simulink model "Mmc"  (R2024b)
settings: Solver=ode23t  StartTime=0.0  StopTime=1  FixedStep=Ts_Power
values from neighbouring files (symbols this model uses):
  C_PM = 8e5    (= 800000)    [MmcParameters.m]    (also in MmcParameters_GFL.m = 0.006)
  Fnom = 50    [MmcParameters.m]    (also in MmcParameters_GFL.m)
  I_b = Snom/Vnom_AC/sqrt(3)    [MmcParameters.m]    (also in MmcParameters_GFL.m)
  Ipp_b = Snom/Vnom_AC/sqrt(3/2)    [MmcParameters.m]    (also in MmcParameters_GFL.m)
  kicir = R0*alpha_i    (= 17453.2925199)    [MmcParameters.m]    (also in MmcParameters_GFL.m = 523.598775598)
  kiout = R*alpha_i    (= 8726.64625997)    [MmcParameters.m]    (also in MmcParameters_GFL.m = 1308.996939)
  kip = alpha_p    (= 34906.5850399)    [MmcParameters.m]    (also in MmcParameters_GFL.m = 100)
  kpcir = L0*alpha_i    (= 2688.88888889)    [MmcParameters.m]    (also in MmcParameters_GFL.m = 66.6666666667)
  kpout = L*alpha_i    (= 1344.44444444)    [MmcParameters.m]    (also in MmcParameters_GFL.m = 166.666666667)
  kpp = alpha_p / alpha_i    (= 0.2)    [MmcParameters.m]    (also in MmcParameters_GFL.m = 0.00381971863421)
  L = L0/2    (= 0.00770309924565)    [MmcParameters.m]    (also in MmcParameters_GFL.m = 0.00636619772368)
  L0 = .2 * L_b    (= 0.0154061984913)    [MmcParameters.m]    (also in MmcParameters_GFL.m = 0.0127323954474)
  Lac = 32e-3    (= 0.032)    [MmcParameters.m]
  Nb_PM = 20    [MmcParameters.m]    (also in MmcParameters_GFL.m)
  R0 = .1    (= 0.1)    [MmcParameters.m]    (also in MmcParameters_GFL.m)
  Rac = 1    [MmcParameters.m]
  SCR = 2    [MmcParameters_GFL.m]
  SigmaM = 10    [MmcParameters_GFL.m]
  Snom = 80e6    (= 80000000)    [MmcParameters.m]    (also in MmcParameters_GFL.m)
  Ts_Power = 2e-6    (= 2e-06)    [MmcParameters.m]    (also in MmcParameters_GFL.m = 1e-05)
  V_b = Vnom_AC    (= 44000)    [MmcParameters.m]    (also in MmcParameters_GFL.m = 40000)
  VDCm = 80e3    (= 80000)    [MmcParameters.m]    (also in MmcParameters_GFL.m = 48000)
  VDCp = 80e3    (= 80000)    [MmcParameters.m]    (also in MmcParameters_GFL.m = 48000)
  Vnom_AC = 44e3    (= 44000)    [MmcParameters.m]    (also in MmcParameters_GFL.m = 40000)
  Vnom_PM = 4e3    (= 4000)    [MmcParameters.m]    (also in MmcParameters_GFL.m = 4800)
  w_b = 2*pi*Fnom    (= 314.159265359)    [MmcParameters.m]    (also in MmcParameters_GFL.m)
libraries: spsSeriesRLCBranchLib x8, spsCurrentMeasurementLib x7, spsHalfBridgeMMCLib x6, slpidlib x6, spsMeanLib x3, spsabctodq0Lib x3, spsDCVoltageSourceLib x2, spsdq0toabcLib x2, spsGroundLib x1, spsThreePhaseVIMeasurementLib x1, spsPLL3phLib x1, spsVoltageMeasurementLib x1
(part 1 of 2)
settings Model: Creator=The MathWorks, Inc.  LastModifiedBy=smile
settings SolverCC: AlgebraicLoopSolver=TrustRegion
settings DataIOCC: SaveFormat=StructureWithTime  SaveOutput=off  SignalLogging=off  DSMLogging=off  SaveTime=off  ReturnWorkspaceOutputs=off
settings OptimizationCC: ExpressionDepthLimit=2147483647  LifeSpan=inf
settings DebuggingCC: UnderspecifiedInitializationDetection=Classic  MergeDetectMultiDrivingBlocksExec=none  SolverPrmCheckMsg=warning  FcnCallInpInsideContextMsg=warning  UnconnectedInputMsg=warning  UnconnectedOutputMsg=warning  UnconnectedLineMsg=warning  AllowSymbolicDim=off  StateNameClashWarn=warning  SFUnexpectedBacktrackingDiag=warning  SFNoUnconditionalDefaultTransitionDiag=warning  SFExecutionAtInitializationDiag=none  ArithmeticOperatorsInVariantConditions=warning
settings HardwareCC: ProdBitPerPointer=32  ProdBitPerSizeT=32  ProdBitPerPtrDiffT=32  ProdLargestAtomicFloat=None  ProdIntDivRoundTo=Undefined  ProdEndianess=Unspecified  ProdWordSize=32  ProdHWDeviceType=32-bit Generic
settings ModelReferenceCC: EnableRefExpFcnMdlSchedulingChecks=on  PropagateSignalLabelsOutOfModel=off
settings SFSimCC: SimUseLocalCustomCode=off  CustomCodeUndefinedFunction=UseInterfaceOnly
settings RTWCC: RTWUseLocalCustomCode=off  GPUComputeCapability=3.5
settings CodeAppCC: StateflowObjectComments=on
settings GRTTargetCC: TargetLangStandard=C89/C90 (ANSI)  CombineOutputUpdateFcns=off  GRTInterface=on
settings ConfigComp: CovMetricSettings=dw  CovSaveCumulativeToWorkspaceVar=on  CovSaveSingleToWorkspaceVar=on  CovExternalEMLEnable=off
settings SimscapeCC: SimscapeNormalizeSystem=off  SimscapeNominalValues={1, 'bar'; 1, 'cm^3/s'; 1, 'bar*kg/s'; 1, 'kJ/kg'; 1, 'kW'; }

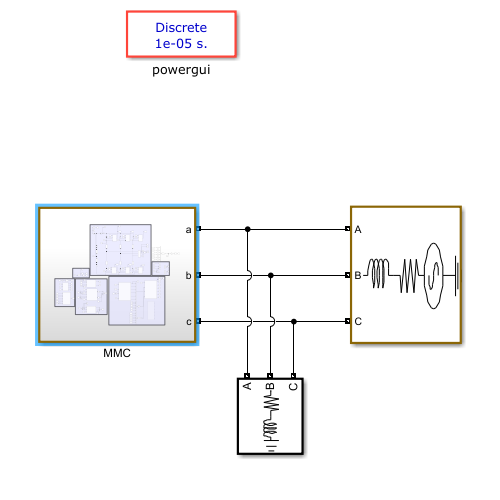
[thumbnail: Simulink's stored preview of the top-level diagram]
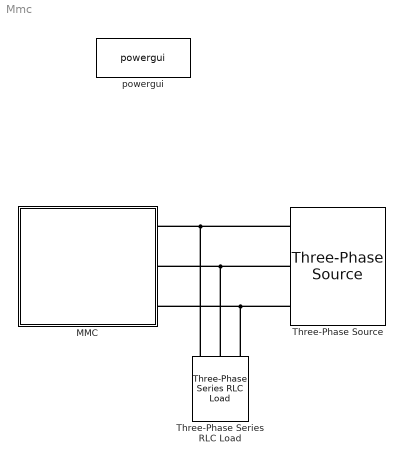
== system Mmc ==
  MMC : Subsystem
  Three-Phase Series RLC Load : spsThreePhaseSeriesRLCLoadLib/Three-Phase Series RLC Load  LConnTagsString=A|B|C  Configuration=Y (grounded)  NominalVoltage=Vnom_AC  Vabc=[1e3 1e3 1e3]  Vabcp=[1e3 1e3 1e3]  NominalFrequency=Fnom  UnbalancedPower=off  ActivePower=Snom/2  InductivePower=Snom/2  CapacitivePower=0  Pabc=[10e3 9e3 11e3]  QLabc=[100 90 110]  QCabc=[100 90 110]  Pabcp=[10e3 9e3 11e3]  QLabcp=[100 90 110]  QCabcp=[100 90 110]  Measurements=None  LoadType=constant Z
  Three-Phase Source : spsThreePhaseSourceLib/Three-Phase Source  InternalConnection=Yg  VoltagePhases=off  Voltage=Vnom_AC  PhaseAngle=0  Voltage_phases=[25e3 25e3 25e3]/sqrt(3)  PhaseAngles_phases=[0 -120 +120]  Frequency=50  NonIdealSource=on  SpecifyImpedance=on  Resistance=Rac/1e9  Inductance=Lac/1e4  ShortCircuitLevel=SCR*Snom  BaseVoltage=Vnom_AC  XRratio=7  BusType=swing  Pref=10e3  Qref=0  Prefabc=[10e3, 10e3, 10e3]  Qrefabc=[0, 0, 0]  Qmin=-inf  Qmax=inf
  powergui : sps_lib/powergui  Priority=1  SimulationMode=Discrete  SampleTime=Ts_Power  frequency=60  Iterations=50  frequencyindice=0  Pbase=100e6  ErrMax=1e-4  UnitsV=kV  UnitsW=MW  buscounter=0  FunctionMessages=off  echomessages=off  EnableUseOfTLC=off  CurrentSourceSwitches=off  DisableSnubberDevices=off  DisableRonSwitches=off  DisableVfSwitches=off  DisplayEquations=off  AutomaticDiscreteSolvers=off  SolverType=Tustin/Backward Euler (TBE)  Interpol=off  ExternalGateDelay=off  methode=off  Ts=10  x0status=blocks  SPID=off  SwTol=0  HookPort=off  NonlinearTolerance=1e-4  nMaxIteration=100  ContinueOnMaxIteration=off  RestoreLinks=warning  ResistiveCurrentMeasurement=off  Frange=[0:2:500]  Ylog=off  Xlog=on  ShowGrid=off  save=off  variable=ZData  structure=Vout  ZoomFFT=on  StartTime=0.15  cycles=2  DisplayStyle=1  fundamental=50  FreqAxis=on  MaxFrequency=6000  frequencyindicesteady=1  RmsSteady=1  display=off
  connections:
  Three-Phase Source/RConn1 -- Three-Phase Series RLC Load/LConn1 -- MMC/LConn1
  Three-Phase Source/RConn2 -- Three-Phase Series RLC Load/LConn2 -- MMC/LConn2
  Three-Phase Source/RConn3 -- Three-Phase Series RLC Load/LConn3 -- MMC/LConn3

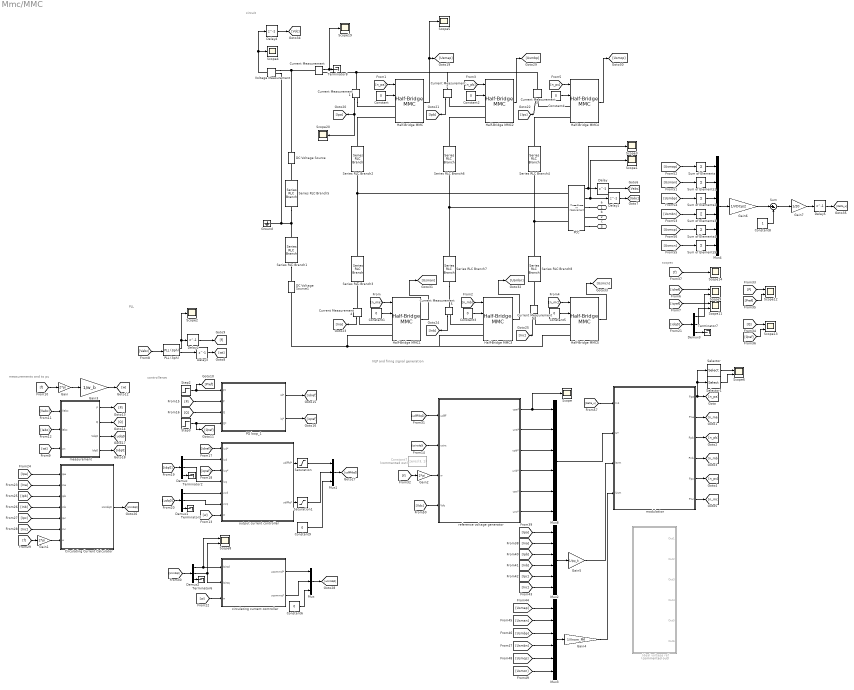
== system Mmc/MMC ==
  note: controllerws
  note: circuit
  note: scopes
  note: NLP and firing signal generation
  note: measurements and to pu
  note: PLL
  Circulating Current Calculator : Subsystem
  Constant{,1..6,9} (8 alike) : Constant  Value=0
  Constant7 : Constant  Commented=on  Value=zeros(3, 1)
  Constant8 : Constant
  Current Measurement{,1..6} (7 alike) : spsCurrentMeasurementLib/Current Measurement  PhasorSimulation=off  OutputType=Complex  PSBequivalent=0
  DC Voltage Source : spsDCVoltageSourceLib/DC Voltage Source  Amplitude=VDCp  Measurements=None
  DC Voltage Source1 : spsDCVoltageSourceLib/DC Voltage Source  Amplitude=VDCm  Measurements=None
  Delay{,1..3} (4 alike) : Delay  DelayLength=1  SampleTime=Ts_Power
  Delay4 : Delay  DelayLength=1  InputProcessing=Columns as channels (frame based)
  Delay5 : Delay  DelayLength=1  InputProcessing=Columns as channels (frame based)  SampleTime=Ts_Power
  Demux{,1..3} (4 alike) : Demux  Outputs=3
  Gain : Gain  Gain=2*pi
  Gain1 : Gain  Gain=2*pi
  Gain2 : Gain  Gain=2*pi
  Gain3 : Gain  Gain=1/w_b
  Gain4 : Gain  Gain=1/Vnom_PM
  Gain5 : Gain  Gain=1/Ipp_b
  Gain6 : Gain  Gain=1/VDCp/2
  Gain7 : Gain  Gain=1/20
  Ground : spsGroundLib/Ground  LConnTagsString=a
  Half-Bridge MMC{,1..5} (6 alike) : spsHalfBridgeMMCLib/Half-Bridge MMC  ModelType=Switching devices  n=Nb_PM  C=C_PM  Vc_Initial=Vc_Initial  Ron=Ron  Rs=Rs  Cs=Cs  Ron_Diode=1e-3  Rs_Diode=1e6  Cs_Diode=inf  Vf_Diode=1e-3  Rs_CurrentSource=inf  Ts=10e-6
      settings: LibrarySourceBlock=sps_lib/Power Electronics/Half-Bridge MMC
  Ideal voltage ref : Subsystem  Commented=on
  Mux : Mux  Inputs=3
  Mux1 : Mux  Inputs=3
  Mux{2..4,8} (4 alike) : Mux  Inputs=6
  PCC : spsThreePhaseVIMeasurementLib/Three-Phase V-I Measurement  VoltageMeasurement=phase-to-ground  SetLabelV=off  LabelV=Vabc  Vpu=on  VpuLL=off  CurrentMeasurement=yes  SetLabelI=off  LabelI=Iabc  Ipu=on  Pbase=Snom  Vbase=Vnom_AC  OutputType=Complex  PhasorSimulation=off  PSBequivalent=0
  PLL (3ph) : spsPLL3phLib/PLL (3ph)  Fmin=45  Par_Init=[0, 50]  ParK=[9.2/.2 (4.6/.2/.7)^2 0]  TcD=1e-4  MaxRateChangeFreq=12  FilterCutOffFreq=50  Ts=0  AGC=on
  PQ loop_1 : Subsystem
  Saturation : Saturate  UpperLimit=1.2  LowerLimit=-1.2
  Saturation1 : Saturate  UpperLimit=1.2  LowerLimit=-1.2
  Scope{,1..5,14,19..20} (9 alike) : Scope
  Scope{6,8..9,11..13} (6 alike) : Scope  NumInputPorts=2
  Selector : Selector  InputPortWidth=2*Nb_PM  IndexOptions=Index vector (dialog)  Indices=[1]  OutputSizes=1
  Selector1 : Selector  InputPortWidth=2*Nb_PM  IndexOptions=Index vector (dialog)  Indices=[Nb_PM]  OutputSizes=1
  Series RLC Branch{1..8} (8 alike) : spsSeriesRLCBranchLib/Series RLC Branch  LConnTagsString=__new0  RConnTagsString=__new0  BranchType=RL  Resistance=R0  Inductance=L0  SetiL0=off  InitialCurrent=0  Capacitance=1e-6  Setx0=off  InitialVoltage=0  Measurements=None
  Step2 : Step  Time=.3  Before=-.1  After=.7  SampleTime=Ts_Power
  Step3 : Step  Time=.7  Before=-.1  After=0.7  SampleTime=Ts_Power
  Sum : Sum  Inputs=|+-
  Sum of Elements{,1..5} (6 alike) : Sum  Inputs=+
  Terminator{2..3,6..8} (5 alike) : Terminator
  Voltage Measurement : spsVoltageMeasurementLib/Voltage Measurement  PhasorSimulation=off  OutputType=Complex  PSBequivalent=0
  circulating current controller : Subsystem
  measurement : Subsystem
  modulation : Subsystem
  output current controller : Subsystem
  reference voltage generator : Subsystem
  a : PMIOPort  Side=Left
  b : PMIOPort  Port=2  Side=Left
  c : PMIOPort  Port=3  Side=Left
  wires:
  Constant4/1 -> Half-Bridge MMC4/2
  [n_pc] -> Half-Bridge MMC4/1
  [n_pb] -> Half-Bridge MMC2/1
  [n_pa] -> Half-Bridge MMC/1
  [n_mb] -> Half-Bridge MMC3/1
  Constant1/1 -> Half-Bridge MMC1/2
  Constant3/1 -> Half-Bridge MMC3/2
  Half-Bridge MMC/1 -> Scope5/1, [Usmap]
  Constant2/1 -> Half-Bridge MMC2/2
  Constant/1 -> Half-Bridge MMC/2
  [n_ma] -> Half-Bridge MMC1/1
  Constant5/1 -> Half-Bridge MMC5/2
  [n_mc] -> Half-Bridge MMC5/1
  PCC/1 -> Scope3/1, Delay/1
  PCC/2 -> Scope1/1, Delay1/1
  [Vabc] -> measurement/1(Vabc)
  [Iabc] -> measurement/2(Iabc)
  [Vabc] -> PLL (3ph)/1
  PLL (3ph)/2 -> Delay3/1
  [wt] -> measurement/3(wt)
  PLL (3ph)/1 -> Scope2/1, Delay2/1
  [f] -> Gain/1
  Gain/1 -> Gain3/1
  Gain3/1 -> [w]
  [w] -> output current controller/7(w)
  circulating current controller/1(ucommd*) -> Mux/1
  circulating current controller/2(ucommq*) -> Mux/2
  Constant6/1 -> Mux/3
  measurement/1(P) -> [P]
  [idref] -> output current controller/1(ivd*)
  [iqref] -> output current controller/3(ivq*)
  measurement/3(Vdq0) -> [udq0]
  measurement/4(Idq0) -> [idq0]
  [idq0] -> Demux/1
  Demux/2 -> output current controller/4(ivq)
  Demux/1 -> output current controller/2(ivd)
  Demux/3 -> Terminator2/1
  [udq0] -> Demux1/1
  Demux1/1 -> output current controller/5(uvd)
  Demux1/2 -> output current controller/6(uvq)
  Demux1/3 -> Terminator3/1
  [w] -> circulating current controller/3(w)
  Current Measurement1/1 -> Scope20/1, [Ipa]
  Current Measurement2/1 -> [Ipb]
  Current Measurement3/1 -> [Ipc]
  Current Measurement4/1 -> [Ina]
  Current Measurement5/1 -> [Inb]
  Current Measurement6/1 -> [Inc]
  [Ipa] -> Circulating Current Calculator/1(ipa)
  [Ina] -> Circulating Current Calculator/2(ina)
  [Ipb] -> Circulating Current Calculator/3(ipb)
  [Inb] -> Circulating Current Calculator/4(inb)
  [Ipc] -> Circulating Current Calculator/5(ipc)
  [Inc] -> Circulating Current Calculator/6(inc)
  [f] -> Gain1/1
  Gain1/1 -> Circulating Current Calculator/7(w)
  Circulating Current Calculator/1(icircdq0) -> [Icircdq0]
  [Icircdq0] -> Demux2/1
  Demux2/1 -> Scope8/1, circulating current controller/1(Icircd)
  Demux2/2 -> circulating current controller/2(Icircq), Scope8/2
  Demux2/3 -> Terminator6/1
  Constant9/1 -> Mux1/3
  Mux1/1 -> [udiffdq0]
  Gain2/1 -> reference voltage generator/3(w)
  [f] -> Gain2/1
  measurement/2(Q) -> [Q]
  Step3/1 -> PQ loop_1/4(Q*), [Qref]
  Delay/1 -> [Vabc]
  Delay1/1 -> [Iabc]
  Delay2/1 -> [f]
  Delay3/1 -> [wt]
  modulation/1(Ppa) -> [n_pa], Selector1/1, Selector/1
  modulation/2(Pna) -> [n_ma]
  modulation/3(Ppb) -> [n_pb]
  modulation/4(Pnb) -> [n_mb]
  modulation/5(Ppc) -> [n_pc]
  modulation/6(Pnc) -> [n_mc]
  output current controller/1(udiffd*) -> Saturation/1
  Saturation/1 -> Mux1/1
  output current controller/2(udiffq*) -> Saturation1/1
  Saturation1/1 -> Mux1/2
  Step2/1 -> PQ loop_1/1(P*), [Pref]
  PQ loop_1/1(id*) -> [idref]
  PQ loop_1/2(iq*) -> [iqref]
  [idq0] -> Demux3/1
  Demux3/3 -> Terminator7/1
  [idref] -> Scope9/1
  Demux3/1 -> Scope9/2
  [iqref] -> Scope11/1
  Demux3/2 -> Scope11/2
  Mux/1 -> [ucircdq0]
  [P] -> Scope12/1
  [Pref] -> Scope12/2
  [Q] -> Scope13/1
  [Qref] -> Scope13/2
  [f] -> Scope14/1
  [P] -> PQ loop_1/2(P)
  [Q] -> PQ loop_1/3(Q)
  [udiffdq0] -> reference voltage generator/1(udiff)
  reference voltage generator/1(upa*) -> Scope/1, Mux8/1
  reference voltage generator/2(una*) -> Mux8/2
  reference voltage generator/3(upb*) -> Mux8/3
  reference voltage generator/4(unb*) -> Mux8/4
  reference voltage generator/5(upc*) -> Mux8/5
  reference voltage generator/6(unc*) -> Mux8/6
  [Ipa] -> Mux2/1
  [Ina] -> Mux2/2
  [Ipb] -> Mux2/3
  [Inb] -> Mux2/4
  [Ipc] -> Mux2/5
  [Inc] -> Mux2/6
  Mux2/1 -> Gain5/1
  Current Measurement/1 -> Scope19/1, Terminator8/1
  Half-Bridge MMC2/1 -> [Usmbp]
  Half-Bridge MMC4/1 -> [Usmcp]
  Half-Bridge MMC1/1 -> [Usman]
  Half-Bridge MMC3/1 -> [Usmbn]
  Half-Bridge MMC5/1 -> [Usmcn]
  [Usmap] -> Mux3/1
  [Usman] -> Mux3/2
  [Usmbp] -> Mux3/3
  [Usmbn] -> Mux3/4
  [Usmcp] -> Mux3/5
  Mux3/1 -> Gain4/1
  [Usmcn] -> Mux3/6
  Gain4/1 -> modulation/4(Usm)
  Gain5/1 -> modulation/3(Iarm)
  Selector/1 -> Scope6/1
  Selector1/1 -> Scope6/2
  Voltage Measurement/1 -> Delay4/1, Scope4/1
  Delay4/1 -> [Vdc]
  Mux8/1 -> modulation/2(U*)
  [Vdc] -> reference voltage generator/4(Vdc)
  [Usmap] -> Sum of Elements/1
  [Usman] -> Sum of Elements1/1
  [Usmbn] -> Sum of Elements3/1
  [Usmbp] -> Sum of Elements2/1
  [Usmcp] -> Sum of Elements4/1
  [Usmcn] -> Sum of Elements5/1
  Sum of Elements/1 -> Mux4/1
  Sum of Elements1/1 -> Mux4/2
  Sum of Elements2/1 -> Mux4/3
  Sum of Elements3/1 -> Mux4/4
  Sum of Elements4/1 -> Mux4/5
  Sum of Elements5/1 -> Mux4/6
  [Delta_u] -> modulation/1(In1)
  Mux4/1 -> Gain6/1
  Constant8/1 -> Sum/2
  Delay5/1 -> [Delta_u]
  Gain6/1 -> Sum/1
  Gain7/1 -> Delay5/1
  [ucircdq0] -> reference voltage generator/2(ucirc)
  Sum/1 -> Gain7/1
  connections:
  Series RLC Branch1/RConn1 -- DC Voltage Source1/RConn1
  Half-Bridge MMC5/LConn2 -- Half-Bridge MMC3/LConn2 -- Half-Bridge MMC1/LConn2 -- DC Voltage Source1/LConn1
  Series RLC Branch4/LConn1 -- Half-Bridge MMC4/LConn2
  Current Measurement/RConn1 -- Current Measurement2/LConn1 -- Current Measurement3/LConn1 -- Current Measurement1/LConn1
  Series RLC Branch8/LConn1 -- PCC/LConn3 -- Series RLC Branch4/RConn1
  Series RLC Branch1/LConn1 -- Series RLC Branch5/RConn1 -- Voltage Measurement/LConn2 -- Ground/LConn1
  Series RLC Branch2/LConn1 -- Half-Bridge MMC/LConn2
  Series RLC Branch3/LConn1 -- Series RLC Branch2/RConn1 -- PCC/LConn1
  Series RLC Branch6/LConn1 -- Half-Bridge MMC2/LConn2
  Series RLC Branch7/LConn1 -- Series RLC Branch6/RConn1 -- PCC/LConn2
  Series RLC Branch5/LConn1 -- DC Voltage Source/LConn1
  PCC/RConn1 -- a/RConn1
  b/RConn1 -- PCC/RConn2
  PCC/RConn3 -- c/RConn1
  Current Measurement/LConn1 -- DC Voltage Source/RConn1 -- Voltage Measurement/LConn1
  Current Measurement1/RConn1 -- Half-Bridge MMC/LConn1
  Half-Bridge MMC2/LConn1 -- Current Measurement2/RConn1
  Half-Bridge MMC4/LConn1 -- Current Measurement3/RConn1
  Half-Bridge MMC1/LConn1 -- Current Measurement4/RConn1
  Current Measurement4/LConn1 -- Series RLC Branch3/RConn1
  Series RLC Branch7/RConn1 -- Current Measurement5/LConn1
  Half-Bridge MMC3/LConn1 -- Current Measurement5/RConn1
  Current Measurement6/LConn1 -- Series RLC Branch8/RConn1
  Half-Bridge MMC5/LConn1 -- Current Measurement6/RConn1

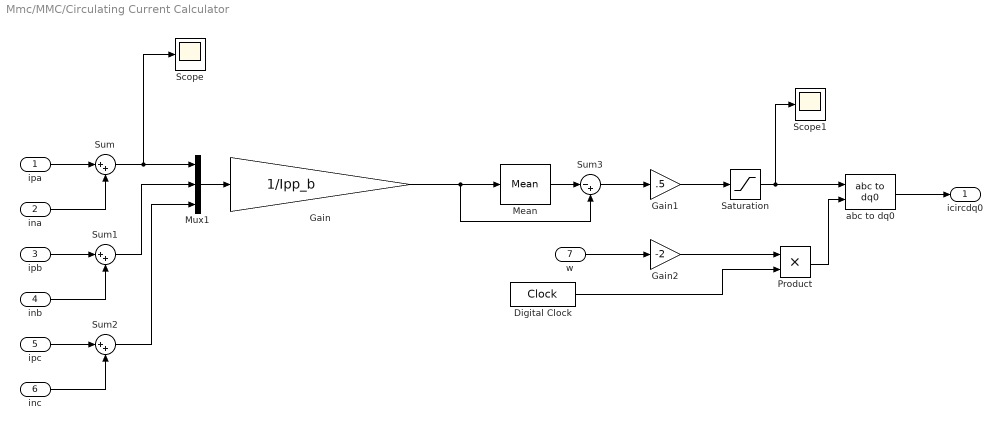
== system Mmc/MMC/Circulating Current Calculator ==
  ipa : Inport
  ina : Inport  Port=2
  ipb : Inport  Port=3
  inb : Inport  Port=4
  ipc : Inport  Port=5
  inc : Inport  Port=6
  w : Inport  Port=7
  Digital Clock : DigitalClock  SampleTime=Ts_Power
  Gain : Gain  Gain=1/Ipp_b
  Gain1 : Gain  Gain=.5
  Gain2 : Gain  Gain=-2
  Mean : spsMeanLib/Mean  Freq=Fnom*2*2  Vinit=0  Ts=Ts_Power
  Mux1 : Mux  Inputs=3
  Product : Product
  Saturation : Saturate  UpperLimit=1.2  LowerLimit=-1.2
  Scope : Scope
  Scope1 : Scope
  Sum : Sum  Inputs=|++
  Sum1 : Sum  Inputs=|++
  Sum2 : Sum  Inputs=|++
  Sum3 : Sum  Inputs=|-+
  abc to dq0 : spsabctodq0Lib/abc to dq0  Alignment=90 degrees behind phase A axis
  icircdq0 : Outport
  wires:
  Sum2/1 -> Mux1/3
  ina/1 -> Sum/2
  Mux1/1 -> Gain/1
  ipb/1 -> Sum1/1
  Sum/1 -> Scope/1, Mux1/1
  Sum1/1 -> Mux1/2
  ipc/1 -> Sum2/1
  inb/1 -> Sum1/2
  ipa/1 -> Sum/1
  inc/1 -> Sum2/2
  Gain1/1 -> Saturation/1
  abc to dq0/1 -> icircdq0/1
  w/1 -> Gain2/1
  Gain2/1 -> Product/1
  Digital Clock/1 -> Product/2
  Product/1 -> abc to dq0/2
  Mean/1 -> Sum3/1
  Sum3/1 -> Gain1/1
  Gain/1 -> Mean/1, Sum3/2
  Saturation/1 -> Scope1/1, abc to dq0/1

== system Mmc/MMC/Ideal voltage ref ==
  Gain4 : Gain  Gain=-1
  Gain5 : Gain  Gain=-1
  Gain6 : Gain  Gain=-1
  Sine Wave : Sin  Amplitude=sqrt(3/2)  Frequency=50*2*pi  SampleTime=Ts_Power
  Sine Wave1 : Sin  Amplitude=Vnom_AC*sqrt(2/3)/Vnom_PM/Nb_PM  Frequency=50*2*pi  Phase=4*pi/3  SampleTime=Ts_Power
  Sine Wave2 : Sin  Amplitude=Vnom_AC*sqrt(2/3)/Vnom_PM/Nb_PM  Frequency=50*2*pi  Phase=2*pi/3  SampleTime=Ts_Power
  Out1 : Outport
  Out2 : Outport  Port=2
  Out3 : Outport  Port=3
  Out4 : Outport  Port=4
  Out5 : Outport  Port=5
  Out6 : Outport  Port=6
  wires:
  Gain4/1 -> Out2/1
  Sine Wave1/1 -> Out3/1, Gain5/1
  Sine Wave2/1 -> Out5/1, Gain6/1
  Sine Wave/1 -> Out1/1, Gain4/1
  Gain6/1 -> Out6/1
  Gain5/1 -> Out4/1

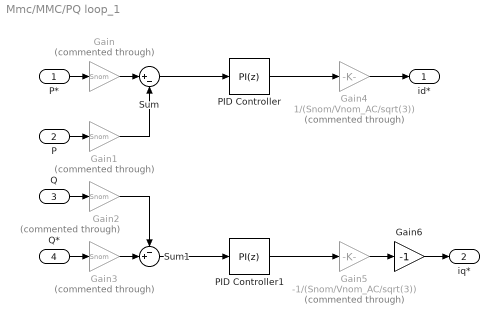
== system Mmc/MMC/PQ loop_1 ==
  P* : Inport
  P : Inport  Port=2
  Q : Inport  Port=3
  Q* : Inport  Port=4
  Gain{,1..3} (4 alike) : Gain  Commented=through  Gain=Snom
  Gain4 : Gain  Commented=through  Gain=1/(Snom/Vnom_AC/sqrt(3))
  Gain5 : Gain  Commented=through  Gain=-1/(Snom/Vnom_AC/sqrt(3))
  Gain6 : Gain  Gain=-1
  PID Controller : slpidlib/PID Controller  Controller=PI  Form=Parallel  TimeDomain=Discrete-time  UseExternalTs=off  SampleTime=-1  IntegratorMethod=Forward Euler  FilterMethod=Forward Euler  ControllerParametersSource=internal  P=kpp  I=kip  UseKiTs=off  D=0  UseExternalDerivativeSource=off  N=100  UseFilter=on  TunerSelectOption=Transfer Function Based (PID Tuner App)  InitialConditionSource=internal  InitialConditionForIntegrator=0  InitialConditionForFilter=0  DifferentiatorICPrevScaledInput=0  ExternalReset=none  TrackingMode=off  Kt=1  LimitOutput=off  SatLimitsSource=internal  UpperSaturationLimit=inf  LowerSaturationLimit=-inf  LinearizeAsGain=on  AntiWindupMode=none  Kb=1  LimitIntegrator=off  UpperIntegratorSaturationLimit=inf  LowerIntegratorSaturationLimit=-inf  POutMin=[]  POutMax=[]  IOutMin=[]  IOutMax=[]  DOutMin=[]  DOutMax=[]  NOutMin=[]  NOutMax=[]  SumOutMin=[]  SumOutMax=[]  SaturationOutMin=[]  SaturationOutMax=[]  PParamMin=[]  PParamMax=[]  IParamMin=[]  IParamMax=[]  DParamMin=[]  DParamMax=[]  NParamMin=[]  NParamMax=[]  KbParamMin=[]  KbParamMax=[]  KtParamMin=[]  KtParamMax=[]  KbOutMin=[]  KbOutMax=[]  KtOutMin=[]  KtOutMax=[]  IntegratorOutMin=[]  IntegratorOutMax=[]  FilterOutMin=[]  FilterOutMax=[]  SumI1OutMin=[]  SumI1OutMax=[]  SumI2OutMin=[]  SumI2OutMax=[]  SumI3OutMin=[]  SumI3OutMax=[]  SumI4OutMin=[]  SumI4OutMax=[]  SumDOutMin=[]  SumDOutMax=[]  DifferentiatorOutMin=[]  DifferentiatorOutMax=[]  FilterDiffOutCoefMin=[]  FilterDiffOutCoefMax=[]  ReciprocalOutMin=[]  ReciprocalOutMax=[]  SumDenOutMin=[]  SumDenOutMax=[]  SumNumOutMin=[]  SumNumOutMax=[]  DivideOutMin=[]  DivideOutMax=[]  UdiffTsProdOutMin=[]  UdiffTsProdOutMax=[]  NTsProdOutMin=[]  NTsProdOutMax=[]  UintegralTsProdOutMin=[]  UintegralTsProdOutMax=[]  UngainTsProdOutMin=[]  UngainTsProdOutMax=[]  ClampingZeroOutDataTypeStr=Inherit: Inherit via back propagation  ClampingZeroOutMin=[]  ClampingZeroOutMax=[]  FilterDenConstantOutDataTypeStr=Inherit: Inherit via back propagation  FilterDenConstantOutMin=[]  FilterDenConstantOutMax=[]  PCopyOutDataTypeStr=Inherit: Inherit via back propagation  PCopyOutMin=[]  PCopyOutMax=[]  NCopyOutDataTypeStr=Inherit: Inherit via back propagation  NCopyOutMin=[]  NCopyOutMax=[]  IntegratorContinuousStateAttributes=''  IntegratorStateMustResolveToSignalObject=off  IntegratorRTWStateStorageClass=Auto  FilterContinuousStateAttributes=''  FilterStateMustResolveToSignalObject=off  FilterRTWStateStorageClass=Auto  ParallelPVariant=InternalParameters  IdealPVariant=Disabled  IVariant=InternalParameters  DVariant=Disabled  IntegratorVariant=Discrete  SatVariant=Disabled  AWVariant=Passthrough  PCopyVariant=Disabled  TRVariant=Disabled  FdbkBlocksVariant=Forward  IdealPFdbkVariant=Disabled  SatFdbkVariant=Disabled  DerivativeFilterVariant=Disabled  NVariant=Disabled  NCopyVariant=Disabled_SignalSpec  FilterICVariant=Disabled  IntegratorICVariant=InternalICs  ExternalResetVariant=Disabled  TRSumVariant=Passthrough  SumFdbkVariant=Disabled  SumVariant=Sum_PI  TsampFilterVariant=InternalTs  TsampNgainVariant=Passthrough  TsampIntegralVariant=Disabled_SignalSpec  ExternalSaturationOutDataTypeStr=Inherit: Same as second input  DerivativeSourceVariant=Disabled  PreIntVariant=InternalPreInt
  PID Controller1 : slpidlib/PID Controller  Controller=PI  Form=Parallel  TimeDomain=Discrete-time  UseExternalTs=off  SampleTime=-1  IntegratorMethod=Forward Euler  FilterMethod=Forward Euler  ControllerParametersSource=internal  P=kpp  I=kip  UseKiTs=off  D=0  UseExternalDerivativeSource=off  N=100  UseFilter=on  TunerSelectOption=Transfer Function Based (PID Tuner App)  InitialConditionSource=internal  InitialConditionForIntegrator=0  InitialConditionForFilter=0  DifferentiatorICPrevScaledInput=0  ExternalReset=none  TrackingMode=off  Kt=1  LimitOutput=off  SatLimitsSource=internal  UpperSaturationLimit=inf  LowerSaturationLimit=-inf  LinearizeAsGain=on  AntiWindupMode=none  Kb=1  LimitIntegrator=off  UpperIntegratorSaturationLimit=inf  LowerIntegratorSaturationLimit=-inf  POutMin=[]  POutMax=[]  IOutMin=[]  IOutMax=[]  DOutMin=[]  DOutMax=[]  NOutMin=[]  NOutMax=[]  SumOutMin=[]  SumOutMax=[]  SaturationOutMin=[]  SaturationOutMax=[]  PParamMin=[]  PParamMax=[]  IParamMin=[]  IParamMax=[]  DParamMin=[]  DParamMax=[]  NParamMin=[]  NParamMax=[]  KbParamMin=[]  KbParamMax=[]  KtParamMin=[]  KtParamMax=[]  KbOutMin=[]  KbOutMax=[]  KtOutMin=[]  KtOutMax=[]  IntegratorOutMin=[]  IntegratorOutMax=[]  FilterOutMin=[]  FilterOutMax=[]  SumI1OutMin=[]  SumI1OutMax=[]  SumI2OutMin=[]  SumI2OutMax=[]  SumI3OutMin=[]  SumI3OutMax=[]  SumI4OutMin=[]  SumI4OutMax=[]  SumDOutMin=[]  SumDOutMax=[]  DifferentiatorOutMin=[]  DifferentiatorOutMax=[]  FilterDiffOutCoefMin=[]  FilterDiffOutCoefMax=[]  ReciprocalOutMin=[]  ReciprocalOutMax=[]  SumDenOutMin=[]  SumDenOutMax=[]  SumNumOutMin=[]  SumNumOutMax=[]  DivideOutMin=[]  DivideOutMax=[]  UdiffTsProdOutMin=[]  UdiffTsProdOutMax=[]  NTsProdOutMin=[]  NTsProdOutMax=[]  UintegralTsProdOutMin=[]  UintegralTsProdOutMax=[]  UngainTsProdOutMin=[]  UngainTsProdOutMax=[]  ClampingZeroOutDataTypeStr=Inherit: Inherit via back propagation  ClampingZeroOutMin=[]  ClampingZeroOutMax=[]  FilterDenConstantOutDataTypeStr=Inherit: Inherit via back propagation  FilterDenConstantOutMin=[]  FilterDenConstantOutMax=[]  PCopyOutDataTypeStr=Inherit: Inherit via back propagation  PCopyOutMin=[]  PCopyOutMax=[]  NCopyOutDataTypeStr=Inherit: Inherit via back propagation  NCopyOutMin=[]  NCopyOutMax=[]  IntegratorContinuousStateAttributes=''  IntegratorStateMustResolveToSignalObject=off  IntegratorRTWStateStorageClass=Auto  FilterContinuousStateAttributes=''  FilterStateMustResolveToSignalObject=off  FilterRTWStateStorageClass=Auto  ParallelPVariant=InternalParameters  IdealPVariant=Disabled  IVariant=InternalParameters  DVariant=Disabled  IntegratorVariant=Discrete  SatVariant=Disabled  AWVariant=Passthrough  PCopyVariant=Disabled  TRVariant=Disabled  FdbkBlocksVariant=Forward  IdealPFdbkVariant=Disabled  SatFdbkVariant=Disabled  DerivativeFilterVariant=Disabled  NVariant=Disabled  NCopyVariant=Disabled_SignalSpec  FilterICVariant=Disabled  IntegratorICVariant=InternalICs  ExternalResetVariant=Disabled  TRSumVariant=Passthrough  SumFdbkVariant=Disabled  SumVariant=Sum_PI  TsampFilterVariant=InternalTs  TsampNgainVariant=Passthrough  TsampIntegralVariant=Disabled_SignalSpec  ExternalSaturationOutDataTypeStr=Inherit: Same as second input  DerivativeSourceVariant=Disabled  PreIntVariant=InternalPreInt
  Sum : Sum  Inputs=|+-
  Sum1 : Sum  Inputs=-+|
  id* : Outport
  iq* : Outport  Port=2
  wires:
  P*/1 -> Gain/1
  P/1 -> Gain1/1
  Q*/1 -> Gain3/1
  Q/1 -> Gain2/1
  Sum/1 -> PID Controller/1
  Sum1/1 -> PID Controller1/1
  PID Controller/1 -> Gain4/1
  PID Controller1/1 -> Gain5/1
  Gain/1 -> Sum/1
  Gain1/1 -> Sum/2
  Gain2/1 -> Sum1/1
  Gain3/1 -> Sum1/2
  Gain4/1 -> id*/1
  Gain5/1 -> Gain6/1
  Gain6/1 -> iq*/1

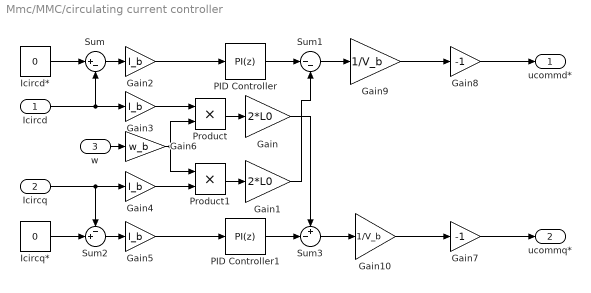
== system Mmc/MMC/circulating current controller ==
  Icircd : Inport
  Icircq : Inport  Port=2
  w : Inport  Port=3
  Gain : Gain  Gain=2*L0
  Gain1 : Gain  Gain=2*L0
  Gain10 : Gain  Gain=1/V_b
  Gain{2..5} (4 alike) : Gain  Gain=I_b
  Gain6 : Gain  Gain=w_b
  Gain7 : Gain  Gain=-1
  Gain8 : Gain  Gain=-1
  Gain9 : Gain  Gain=1/V_b
  Icircd* : Constant  Value=0
  Icircq* : Constant  Value=0
  PID Controller : slpidlib/PID Controller  Controller=PI  Form=Parallel  TimeDomain=Discrete-time  UseExternalTs=off  SampleTime=-1  IntegratorMethod=Forward Euler  FilterMethod=Forward Euler  ControllerParametersSource=internal  P=kpcir  I=kicir  UseKiTs=off  D=0  UseExternalDerivativeSource=off  N=100  UseFilter=on  TunerSelectOption=Transfer Function Based (PID Tuner App)  InitialConditionSource=internal  InitialConditionForIntegrator=0  InitialConditionForFilter=0  DifferentiatorICPrevScaledInput=0  ExternalReset=none  TrackingMode=off  Kt=1  LimitOutput=off  SatLimitsSource=internal  UpperSaturationLimit=inf  LowerSaturationLimit=-inf  LinearizeAsGain=on  AntiWindupMode=none  Kb=1  LimitIntegrator=off  UpperIntegratorSaturationLimit=inf  LowerIntegratorSaturationLimit=-inf  POutMin=[]  POutMax=[]  IOutMin=[]  IOutMax=[]  DOutMin=[]  DOutMax=[]  NOutMin=[]  NOutMax=[]  SumOutMin=[]  SumOutMax=[]  SaturationOutMin=[]  SaturationOutMax=[]  PParamMin=[]  PParamMax=[]  IParamMin=[]  IParamMax=[]  DParamMin=[]  DParamMax=[]  NParamMin=[]  NParamMax=[]  KbParamMin=[]  KbParamMax=[]  KtParamMin=[]  KtParamMax=[]  KbOutMin=[]  KbOutMax=[]  KtOutMin=[]  KtOutMax=[]  IntegratorOutMin=[]  IntegratorOutMax=[]  FilterOutMin=[]  FilterOutMax=[]  SumI1OutMin=[]  SumI1OutMax=[]  SumI2OutMin=[]  SumI2OutMax=[]  SumI3OutMin=[]  SumI3OutMax=[]  SumI4OutMin=[]  SumI4OutMax=[]  SumDOutMin=[]  SumDOutMax=[]  DifferentiatorOutMin=[]  DifferentiatorOutMax=[]  FilterDiffOutCoefMin=[]  FilterDiffOutCoefMax=[]  ReciprocalOutMin=[]  ReciprocalOutMax=[]  SumDenOutMin=[]  SumDenOutMax=[]  SumNumOutMin=[]  SumNumOutMax=[]  DivideOutMin=[]  DivideOutMax=[]  UdiffTsProdOutMin=[]  UdiffTsProdOutMax=[]  NTsProdOutMin=[]  NTsProdOutMax=[]  UintegralTsProdOutMin=[]  UintegralTsProdOutMax=[]  UngainTsProdOutMin=[]  UngainTsProdOutMax=[]  ClampingZeroOutDataTypeStr=Inherit: Inherit via back propagation  ClampingZeroOutMin=[]  ClampingZeroOutMax=[]  FilterDenConstantOutDataTypeStr=Inherit: Inherit via back propagation  FilterDenConstantOutMin=[]  FilterDenConstantOutMax=[]  PCopyOutDataTypeStr=Inherit: Inherit via back propagation  PCopyOutMin=[]  PCopyOutMax=[]  NCopyOutDataTypeStr=Inherit: Inherit via back propagation  NCopyOutMin=[]  NCopyOutMax=[]  IntegratorContinuousStateAttributes=''  IntegratorStateMustResolveToSignalObject=off  IntegratorRTWStateStorageClass=Auto  FilterContinuousStateAttributes=''  FilterStateMustResolveToSignalObject=off  FilterRTWStateStorageClass=Auto  ParallelPVariant=InternalParameters  IdealPVariant=Disabled  IVariant=InternalParameters  DVariant=Disabled  IntegratorVariant=Discrete  SatVariant=Disabled  AWVariant=Passthrough  PCopyVariant=Disabled  TRVariant=Disabled  FdbkBlocksVariant=Forward  IdealPFdbkVariant=Disabled  SatFdbkVariant=Disabled  DerivativeFilterVariant=Disabled  NVariant=Disabled  NCopyVariant=Disabled_SignalSpec  FilterICVariant=Disabled  IntegratorICVariant=InternalICs  ExternalResetVariant=Disabled  TRSumVariant=Passthrough  SumFdbkVariant=Disabled  SumVariant=Sum_PI  TsampFilterVariant=InternalTs  TsampNgainVariant=Passthrough  TsampIntegralVariant=Disabled_SignalSpec  ExternalSaturationOutDataTypeStr=Inherit: Same as second input  DerivativeSourceVariant=Disabled  PreIntVariant=InternalPreInt
  PID Controller1 : slpidlib/PID Controller  Controller=PI  Form=Parallel  TimeDomain=Discrete-time  UseExternalTs=off  SampleTime=-1  IntegratorMethod=Forward Euler  FilterMethod=Forward Euler  ControllerParametersSource=internal  P=kpcir  I=kicir  UseKiTs=off  D=0  UseExternalDerivativeSource=off  N=100  UseFilter=on  TunerSelectOption=Transfer Function Based (PID Tuner App)  InitialConditionSource=internal  InitialConditionForIntegrator=0  InitialConditionForFilter=0  DifferentiatorICPrevScaledInput=0  ExternalReset=none  TrackingMode=off  Kt=1  LimitOutput=off  SatLimitsSource=internal  UpperSaturationLimit=inf  LowerSaturationLimit=-inf  LinearizeAsGain=on  AntiWindupMode=none  Kb=1  LimitIntegrator=off  UpperIntegratorSaturationLimit=inf  LowerIntegratorSaturationLimit=-inf  POutMin=[]  POutMax=[]  IOutMin=[]  IOutMax=[]  DOutMin=[]  DOutMax=[]  NOutMin=[]  NOutMax=[]  SumOutMin=[]  SumOutMax=[]  SaturationOutMin=[]  SaturationOutMax=[]  PParamMin=[]  PParamMax=[]  IParamMin=[]  IParamMax=[]  DParamMin=[]  DParamMax=[]  NParamMin=[]  NParamMax=[]  KbParamMin=[]  KbParamMax=[]  KtParamMin=[]  KtParamMax=[]  KbOutMin=[]  KbOutMax=[]  KtOutMin=[]  KtOutMax=[]  IntegratorOutMin=[]  IntegratorOutMax=[]  FilterOutMin=[]  FilterOutMax=[]  SumI1OutMin=[]  SumI1OutMax=[]  SumI2OutMin=[]  SumI2OutMax=[]  SumI3OutMin=[]  SumI3OutMax=[]  SumI4OutMin=[]  SumI4OutMax=[]  SumDOutMin=[]  SumDOutMax=[]  DifferentiatorOutMin=[]  DifferentiatorOutMax=[]  FilterDiffOutCoefMin=[]  FilterDiffOutCoefMax=[]  ReciprocalOutMin=[]  ReciprocalOutMax=[]  SumDenOutMin=[]  SumDenOutMax=[]  SumNumOutMin=[]  SumNumOutMax=[]  DivideOutMin=[]  DivideOutMax=[]  UdiffTsProdOutMin=[]  UdiffTsProdOutMax=[]  NTsProdOutMin=[]  NTsProdOutMax=[]  UintegralTsProdOutMin=[]  UintegralTsProdOutMax=[]  UngainTsProdOutMin=[]  UngainTsProdOutMax=[]  ClampingZeroOutDataTypeStr=Inherit: Inherit via back propagation  ClampingZeroOutMin=[]  ClampingZeroOutMax=[]  FilterDenConstantOutDataTypeStr=Inherit: Inherit via back propagation  FilterDenConstantOutMin=[]  FilterDenConstantOutMax=[]  PCopyOutDataTypeStr=Inherit: Inherit via back propagation  PCopyOutMin=[]  PCopyOutMax=[]  NCopyOutDataTypeStr=Inherit: Inherit via back propagation  NCopyOutMin=[]  NCopyOutMax=[]  IntegratorContinuousStateAttributes=''  IntegratorStateMustResolveToSignalObject=off  IntegratorRTWStateStorageClass=Auto  FilterContinuousStateAttributes=''  FilterStateMustResolveToSignalObject=off  FilterRTWStateStorageClass=Auto  ParallelPVariant=InternalParameters  IdealPVariant=Disabled  IVariant=InternalParameters  DVariant=Disabled  IntegratorVariant=Discrete  SatVariant=Disabled  AWVariant=Passthrough  PCopyVariant=Disabled  TRVariant=Disabled  FdbkBlocksVariant=Forward  IdealPFdbkVariant=Disabled  SatFdbkVariant=Disabled  DerivativeFilterVariant=Disabled  NVariant=Disabled  NCopyVariant=Disabled_SignalSpec  FilterICVariant=Disabled  IntegratorICVariant=InternalICs  ExternalResetVariant=Disabled  TRSumVariant=Passthrough  SumFdbkVariant=Disabled  SumVariant=Sum_PI  TsampFilterVariant=InternalTs  TsampNgainVariant=Passthrough  TsampIntegralVariant=Disabled_SignalSpec  ExternalSaturationOutDataTypeStr=Inherit: Same as second input  DerivativeSourceVariant=Disabled  PreIntVariant=InternalPreInt
  Product : Product
  Product1 : Product
  Sum : Sum  Inputs=|+-
  Sum1 : Sum  Inputs=|--
  Sum2 : Sum  Inputs=-+|
  Sum3 : Sum  Inputs=+-|
  ucommd* : Outport
  ucommq* : Outport  Port=2
  wires:
  Icircd*/1 -> Sum/1
  Sum/1 -> Gain2/1
  Icircd/1 -> Gain3/1, Sum/2
  Icircq/1 -> Gain4/1, Sum2/1
  Icircq*/1 -> Sum2/2
  Sum2/1 -> Gain5/1
  PID Controller1/1 -> Sum3/2
  PID Controller/1 -> Sum1/1
  w/1 -> Gain6/1
  Product/1 -> Gain/1
  Product1/1 -> Gain1/1
  Sum1/1 -> Gain9/1
  Sum3/1 -> Gain10/1
  Gain/1 -> Sum3/1
  Gain1/1 -> Sum1/2
  Gain2/1 -> PID Controller/1
  Gain3/1 -> Product/1
  Gain6/1 -> Product1/1, Product/2
  Gain4/1 -> Product1/2
  Gain5/1 -> PID Controller1/1
  Gain9/1 -> Gain8/1
  Gain10/1 -> Gain7/1
  Gain8/1 -> ucommd*/1
  Gain7/1 -> ucommq*/1

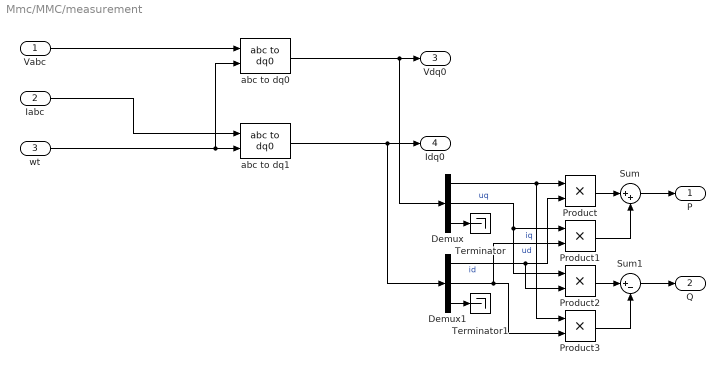
== system Mmc/MMC/measurement ==
  Vabc : Inport
  Iabc : Inport  Port=2
  wt : Inport  Port=3
  Demux : Demux  Outputs=3
  Demux1 : Demux  Outputs=3
  Product{,1..3} (4 alike) : Product
  Sum : Sum  Inputs=|++
  Sum1 : Sum  Inputs=|+-
  Terminator : Terminator
  Terminator1 : Terminator
  abc to dq0 : spsabctodq0Lib/abc to dq0  Alignment=90 degrees behind phase A axis
  abc to dq1 : spsabctodq0Lib/abc to dq0  Alignment=90 degrees behind phase A axis
  P : Outport
  Q : Outport  Port=2
  Vdq0 : Outport  Port=3
  Idq0 : Outport  Port=4
  wires:
  wt/1 -> abc to dq0/2, abc to dq1/2
  Vabc/1 -> abc to dq0/1
  Iabc/1 -> abc to dq1/1
  Demux/3 -> Terminator/1
  Demux1/3 -> Terminator1/1
  Demux/1 -> Product3/1, Product/1  "ud"
  Demux/2 -> Product1/1, Product2/1  "uq"
  Demux1/2 -> Product1/2, Product3/2  "iq"
  Product/1 -> Sum/1
  Product1/1 -> Sum/2
  Product2/1 -> Sum1/1
  Product3/1 -> Sum1/2
  Demux1/1 -> Product2/2, Product/2  "id"
  abc to dq0/1 -> Demux/1, Vdq0/1
  abc to dq1/1 -> Demux1/1, Idq0/1
  Sum/1 -> P/1
  Sum1/1 -> Q/1

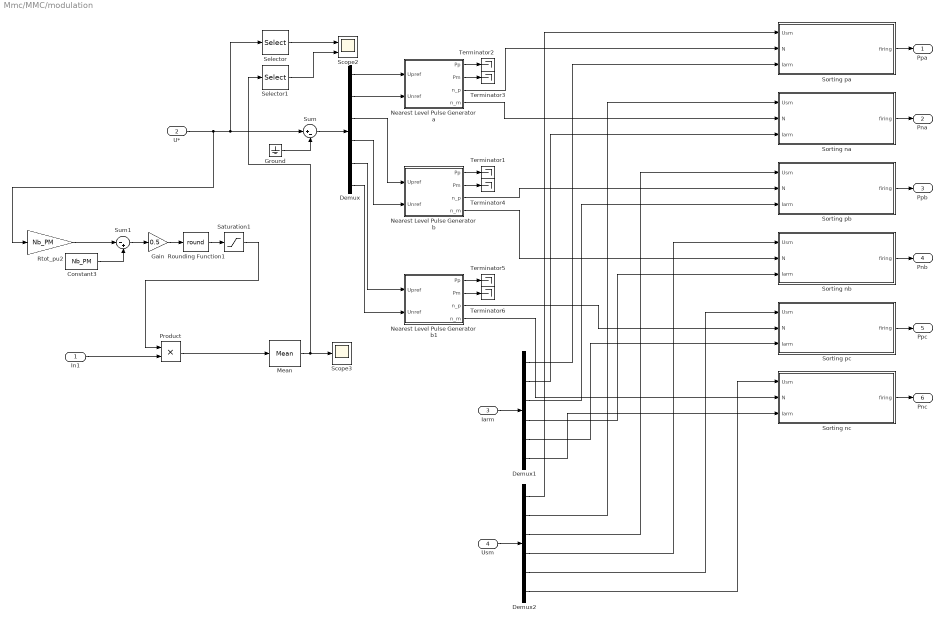
== system Mmc/MMC/modulation ==
  In1 : Inport
  U* : Inport  Port=2
  Iarm : Inport  Port=3
  Usm : Inport  Port=4
  Constant3 : Constant  Value=Nb_PM
  Demux : Demux  Outputs=6
  Demux1 : Demux  Outputs=6
  Demux2 : Demux  Outputs=6
  Gain : Gain  Gain=0.5
  Ground : Ground
  Mean : spsMeanLib/Mean  Freq=Fnom*2  Vinit=0  Ts=Ts_Power
  "Nearest Level Pulse Generator a " : Subsystem
  Nearest Level Pulse Generator b : Subsystem
  Nearest Level Pulse Generator b1 : Subsystem
  Product : Product
  Rounding Function1 : Rounding  Operator=round
  Rtot_pu2 : Gain  Gain=Nb_PM  SaturateOnIntegerOverflow=on  OutDataTypeStr=Inherit: Same as input  ParamDataTypeStr=Inherit: Same as input
  Saturation1 : Saturate  UpperLimit=Nb_PM  LowerLimit=0
  Scope2 : Scope  NumInputPorts=2
  Scope3 : Scope
  Selector : Selector  InputPortWidth=6  IndexOptions=Index vector (dialog)  Indices=[1]  OutputSizes=1
  Selector1 : Selector  InputPortWidth=6  IndexOptions=Index vector (dialog)  Indices=[1]  OutputSizes=1
  Sorting na : Subsystem
  Sorting nb : Subsystem
  Sorting nc : Subsystem
  Sorting pa : Subsystem
  Sorting pb : Subsystem
  Sorting pc : Subsystem
  Sum : Sum  Inputs=|+-
  Sum1 : Sum  Inputs=|-+
  Terminator{1..6} (6 alike) : Terminator
  Ppa : Outport
  Pna : Outport  Port=2
  Ppb : Outport  Port=3
  Pnb : Outport  Port=4
  Ppc : Outport  Port=5
  Pnc : Outport  Port=6
  wires:
  Demux/1 -> "Nearest Level Pulse Generator a "/1(Upref)
  "Nearest Level Pulse Generator a "/3(n_p) -> Sorting pa/2(N)
  "Nearest Level Pulse Generator a "/4(n_m) -> Sorting na/2(N)
  Demux/2 -> "Nearest Level Pulse Generator a "/2(Unref)
  Demux/4 -> Nearest Level Pulse Generator b/2(Unref)
  Demux/3 -> Nearest Level Pulse Generator b/1(Upref)
  Demux/6 -> Nearest Level Pulse Generator b1/2(Unref)
  Demux/5 -> Nearest Level Pulse Generator b1/1(Upref)
  Sorting pa/1(firing) -> Ppa/1
  Sorting na/1(firing) -> Pna/1
  "Nearest Level Pulse Generator a "/1(Pp) -> Terminator2/1
  "Nearest Level Pulse Generator a "/2(Pm) -> Terminator3/1
  Sorting pb/1(firing) -> Ppb/1
  Sorting nb/1(firing) -> Pnb/1
  Nearest Level Pulse Generator b/3(n_p) -> Sorting pb/2(N)
  Nearest Level Pulse Generator b/4(n_m) -> Sorting nb/2(N)
  Nearest Level Pulse Generator b/1(Pp) -> Terminator1/1
  Nearest Level Pulse Generator b/2(Pm) -> Terminator4/1
  Sorting nc/1(firing) -> Pnc/1
  Sorting pc/1(firing) -> Ppc/1
  Nearest Level Pulse Generator b1/3(n_p) -> Sorting pc/2(N)
  Nearest Level Pulse Generator b1/4(n_m) -> Sorting nc/2(N)
  Iarm/1 -> Demux1/1
  Demux1/1 -> Sorting pa/3(Iarm)
  Demux1/2 -> Sorting na/3(Iarm)
  Demux1/3 -> Sorting pb/3(Iarm)
  Demux1/4 -> Sorting nb/3(Iarm)
  Demux1/5 -> Sorting pc/3(Iarm)
  Demux1/6 -> Sorting nc/3(Iarm)
  Usm/1 -> Demux2/1
  Demux2/6 -> Sorting nc/1(Usm)
  Demux2/5 -> Sorting pc/1(Usm)
  Demux2/4 -> Sorting nb/1(Usm)
  Demux2/3 -> Sorting pb/1(Usm)
  Demux2/2 -> Sorting na/1(Usm)
  Demux2/1 -> Sorting pa/1(Usm)
  Nearest Level Pulse Generator b1/1(Pp) -> Terminator5/1
  Nearest Level Pulse Generator b1/2(Pm) -> Terminator6/1
  Sum/1 -> Demux/1
  In1/1 -> Product/2
  Product/1 -> Mean/1
  Mean/1 -> Selector1/1, Scope3/1
  U*/1 -> Rtot_pu2/1, Selector/1, Sum/1
  Sum1/1 -> Gain/1
  Constant3/1 -> Sum1/2
  Gain/1 -> Rounding Function1/1
  Rtot_pu2/1 -> Sum1/1
  Rounding Function1/1 -> Saturation1/1
  Saturation1/1 -> Product/1
  Selector/1 -> Scope2/1
  Selector1/1 -> Scope2/2
  Ground/1 -> Sum/2

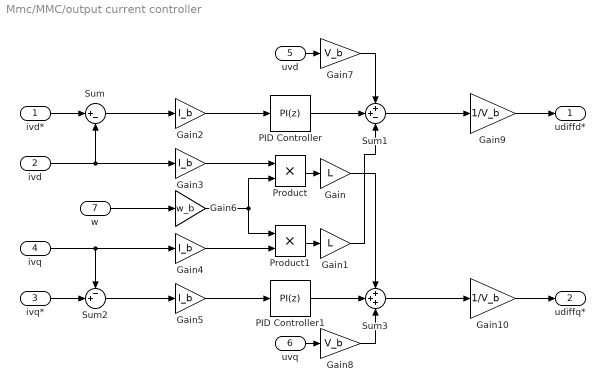
== system Mmc/MMC/output current controller ==
  ivd* : Inport
  ivd : Inport  Port=2
  ivq* : Inport  Port=3
  ivq : Inport  Port=4
  uvd : Inport  Port=5
  uvq : Inport  Port=6
  w : Inport  Port=7
  Gain : Gain  Gain=L
  Gain1 : Gain  Gain=L
  Gain10 : Gain  Gain=1/V_b
  Gain{2..5} (4 alike) : Gain  Gain=I_b
  Gain6 : Gain  Gain=w_b
  Gain7 : Gain  Gain=V_b
  Gain8 : Gain  Gain=V_b
  Gain9 : Gain  Gain=1/V_b
  PID Controller : slpidlib/PID Controller  Controller=PI  Form=Parallel  TimeDomain=Discrete-time  UseExternalTs=off  SampleTime=-1  IntegratorMethod=Forward Euler  FilterMethod=Forward Euler  ControllerParametersSource=internal  P=kpout  I=kiout  UseKiTs=off  D=0  UseExternalDerivativeSource=off  N=100  UseFilter=on  TunerSelectOption=Transfer Function Based (PID Tuner App)  InitialConditionSource=internal  InitialConditionForIntegrator=0  InitialConditionForFilter=0  DifferentiatorICPrevScaledInput=0  ExternalReset=none  TrackingMode=off  Kt=1  LimitOutput=off  SatLimitsSource=internal  UpperSaturationLimit=Vnom_AC  LowerSaturationLimit=-Vnom_AC  LinearizeAsGain=on  AntiWindupMode=clamping  Kb=1  LimitIntegrator=off  UpperIntegratorSaturationLimit=inf  LowerIntegratorSaturationLimit=-inf  POutMin=[]  POutMax=[]  IOutMin=[]  IOutMax=[]  DOutMin=[]  DOutMax=[]  NOutMin=[]  NOutMax=[]  SumOutMin=[]  SumOutMax=[]  SaturationOutMin=[]  SaturationOutMax=[]  PParamMin=[]  PParamMax=[]  IParamMin=[]  IParamMax=[]  DParamMin=[]  DParamMax=[]  NParamMin=[]  NParamMax=[]  KbParamMin=[]  KbParamMax=[]  KtParamMin=[]  KtParamMax=[]  KbOutMin=[]  KbOutMax=[]  KtOutMin=[]  KtOutMax=[]  IntegratorOutMin=[]  IntegratorOutMax=[]  FilterOutMin=[]  FilterOutMax=[]  SumI1OutMin=[]  SumI1OutMax=[]  SumI2OutMin=[]  SumI2OutMax=[]  SumI3OutMin=[]  SumI3OutMax=[]  SumI4OutMin=[]  SumI4OutMax=[]  SumDOutMin=[]  SumDOutMax=[]  DifferentiatorOutMin=[]  DifferentiatorOutMax=[]  FilterDiffOutCoefMin=[]  FilterDiffOutCoefMax=[]  ReciprocalOutMin=[]  ReciprocalOutMax=[]  SumDenOutMin=[]  SumDenOutMax=[]  SumNumOutMin=[]  SumNumOutMax=[]  DivideOutMin=[]  DivideOutMax=[]  UdiffTsProdOutMin=[]  UdiffTsProdOutMax=[]  NTsProdOutMin=[]  NTsProdOutMax=[]  UintegralTsProdOutMin=[]  UintegralTsProdOutMax=[]  UngainTsProdOutMin=[]  UngainTsProdOutMax=[]  ClampingZeroOutDataTypeStr=Inherit: Inherit via back propagation  ClampingZeroOutMin=[]  ClampingZeroOutMax=[]  FilterDenConstantOutDataTypeStr=Inherit: Inherit via back propagation  FilterDenConstantOutMin=[]  FilterDenConstantOutMax=[]  PCopyOutDataTypeStr=Inherit: Inherit via back propagation  PCopyOutMin=[]  PCopyOutMax=[]  NCopyOutDataTypeStr=Inherit: Inherit via back propagation  NCopyOutMin=[]  NCopyOutMax=[]  IntegratorContinuousStateAttributes=''  IntegratorStateMustResolveToSignalObject=off  IntegratorRTWStateStorageClass=Auto  FilterContinuousStateAttributes=''  FilterStateMustResolveToSignalObject=off  FilterRTWStateStorageClass=Auto  ParallelPVariant=InternalParameters  IdealPVariant=Disabled  IVariant=InternalParameters  DVariant=Disabled  IntegratorVariant=Discrete  SatVariant=Disabled  AWVariant=Passthrough  PCopyVariant=Disabled  TRVariant=Disabled  FdbkBlocksVariant=Forward  IdealPFdbkVariant=Disabled  SatFdbkVariant=Disabled  DerivativeFilterVariant=Disabled  NVariant=Disabled  NCopyVariant=Disabled_SignalSpec  FilterICVariant=Disabled  IntegratorICVariant=InternalICs  ExternalResetVariant=Disabled  TRSumVariant=Passthrough  SumFdbkVariant=Disabled  SumVariant=Sum_PI  TsampFilterVariant=InternalTs  TsampNgainVariant=Passthrough  TsampIntegralVariant=Disabled_SignalSpec  ExternalSaturationOutDataTypeStr=Inherit: Same as second input  DerivativeSourceVariant=Disabled  PreIntVariant=InternalPreInt
  PID Controller1 : slpidlib/PID Controller  Controller=PI  Form=Parallel  TimeDomain=Discrete-time  UseExternalTs=off  SampleTime=-1  IntegratorMethod=Forward Euler  FilterMethod=Forward Euler  ControllerParametersSource=internal  P=kpout  I=kiout  UseKiTs=off  D=0  UseExternalDerivativeSource=off  N=100  UseFilter=on  TunerSelectOption=Transfer Function Based (PID Tuner App)  InitialConditionSource=internal  InitialConditionForIntegrator=0  InitialConditionForFilter=0  DifferentiatorICPrevScaledInput=0  ExternalReset=none  TrackingMode=off  Kt=1  LimitOutput=off  SatLimitsSource=internal  UpperSaturationLimit=Vnom_AC  LowerSaturationLimit=-Vnom_AC  LinearizeAsGain=on  AntiWindupMode=clamping  Kb=1  LimitIntegrator=off  UpperIntegratorSaturationLimit=inf  LowerIntegratorSaturationLimit=-inf  POutMin=[]  POutMax=[]  IOutMin=[]  IOutMax=[]  DOutMin=[]  DOutMax=[]  NOutMin=[]  NOutMax=[]  SumOutMin=[]  SumOutMax=[]  SaturationOutMin=[]  SaturationOutMax=[]  PParamMin=[]  PParamMax=[]  IParamMin=[]  IParamMax=[]  DParamMin=[]  DParamMax=[]  NParamMin=[]  NParamMax=[]  KbParamMin=[]  KbParamMax=[]  KtParamMin=[]  KtParamMax=[]  KbOutMin=[]  KbOutMax=[]  KtOutMin=[]  KtOutMax=[]  IntegratorOutMin=[]  IntegratorOutMax=[]  FilterOutMin=[]  FilterOutMax=[]  SumI1OutMin=[]  SumI1OutMax=[]  SumI2OutMin=[]  SumI2OutMax=[]  SumI3OutMin=[]  SumI3OutMax=[]  SumI4OutMin=[]  SumI4OutMax=[]  SumDOutMin=[]  SumDOutMax=[]  DifferentiatorOutMin=[]  DifferentiatorOutMax=[]  FilterDiffOutCoefMin=[]  FilterDiffOutCoefMax=[]  ReciprocalOutMin=[]  ReciprocalOutMax=[]  SumDenOutMin=[]  SumDenOutMax=[]  SumNumOutMin=[]  SumNumOutMax=[]  DivideOutMin=[]  DivideOutMax=[]  UdiffTsProdOutMin=[]  UdiffTsProdOutMax=[]  NTsProdOutMin=[]  NTsProdOutMax=[]  UintegralTsProdOutMin=[]  UintegralTsProdOutMax=[]  UngainTsProdOutMin=[]  UngainTsProdOutMax=[]  ClampingZeroOutDataTypeStr=Inherit: Inherit via back propagation  ClampingZeroOutMin=[]  ClampingZeroOutMax=[]  FilterDenConstantOutDataTypeStr=Inherit: Inherit via back propagation  FilterDenConstantOutMin=[]  FilterDenConstantOutMax=[]  PCopyOutDataTypeStr=Inherit: Inherit via back propagation  PCopyOutMin=[]  PCopyOutMax=[]  NCopyOutDataTypeStr=Inherit: Inherit via back propagation  NCopyOutMin=[]  NCopyOutMax=[]  IntegratorContinuousStateAttributes=''  IntegratorStateMustResolveToSignalObject=off  IntegratorRTWStateStorageClass=Auto  FilterContinuousStateAttributes=''  FilterStateMustResolveToSignalObject=off  FilterRTWStateStorageClass=Auto  ParallelPVariant=InternalParameters  IdealPVariant=Disabled  IVariant=InternalParameters  DVariant=Disabled  IntegratorVariant=Discrete  SatVariant=Disabled  AWVariant=Passthrough  PCopyVariant=Disabled  TRVariant=Disabled  FdbkBlocksVariant=Forward  IdealPFdbkVariant=Disabled  SatFdbkVariant=Disabled  DerivativeFilterVariant=Disabled  NVariant=Disabled  NCopyVariant=Disabled_SignalSpec  FilterICVariant=Disabled  IntegratorICVariant=InternalICs  ExternalResetVariant=Disabled  TRSumVariant=Passthrough  SumFdbkVariant=Disabled  SumVariant=Sum_PI  TsampFilterVariant=InternalTs  TsampNgainVariant=Passthrough  TsampIntegralVariant=Disabled_SignalSpec  ExternalSaturationOutDataTypeStr=Inherit: Same as second input  DerivativeSourceVariant=Disabled  PreIntVariant=InternalPreInt
  Product : Product
  Product1 : Product
  Sum : Sum  Inputs=|+-
  Sum1 : Sum  Inputs=++-
  Sum2 : Sum  Inputs=-+|
  Sum3 : Sum  Inputs=+++
  udiffd* : Outport
  udiffq* : Outport  Port=2
  wires:
  ivd*/1 -> Sum/1
  ivd/1 -> Gain3/1, Sum/2
  Sum/1 -> Gain2/1
  PID Controller/1 -> Sum1/2
  uvd/1 -> Gain7/1
  Sum1/1 -> Gain9/1
  Sum2/1 -> Gain5/1
  PID Controller1/1 -> Sum3/2
  ivq*/1 -> Sum2/2
  ivq/1 -> Sum2/1, Gain4/1
  uvq/1 -> Gain8/1
  Sum3/1 -> Gain10/1
  Product/1 -> Gain/1
  Product1/1 -> Gain1/1
  Gain3/1 -> Product/1
  Gain4/1 -> Product1/2
  Gain5/1 -> PID Controller1/1
  w/1 -> Gain6/1
  Gain6/1 -> Product/2, Product1/1
  Gain9/1 -> udiffd*/1
  Gain10/1 -> udiffq*/1
  Gain7/1 -> Sum1/1
  Gain8/1 -> Sum3/3
  Gain2/1 -> PID Controller/1
  Gain/1 -> Sum3/1
  Gain1/1 -> Sum1/3

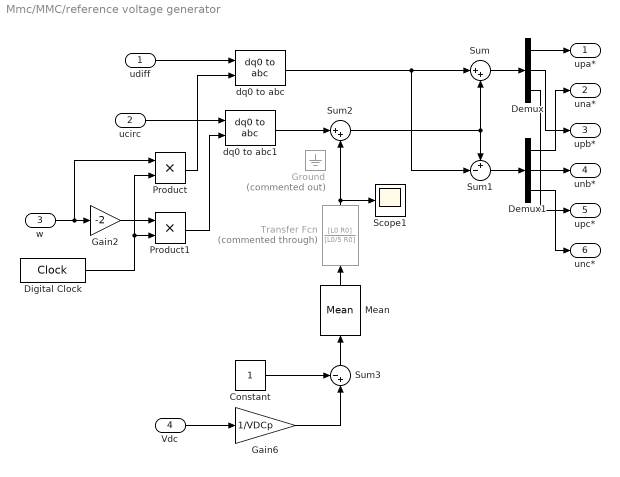
== system Mmc/MMC/reference voltage generator ==
  udiff : Inport
  ucirc : Inport  Port=2
  w : Inport  Port=3
  Vdc : Inport  Port=4
  Constant : Constant
  Demux : Demux  Outputs=3
  Demux1 : Demux  Outputs=3
  Digital Clock : DigitalClock  SampleTime=Ts_Power
  Gain2 : Gain  Gain=-2
  Gain6 : Gain  Gain=1/VDCp
  Ground : Ground  Commented=on
  Mean : spsMeanLib/Mean  Freq=Fnom  Vinit=0  Ts=Ts_Power
  Product : Product
  Product1 : Product
  Scope1 : Scope
  Sum : Sum  Inputs=|++
  Sum1 : Sum  Inputs=+-|
  Sum2 : Sum  Inputs=|++
  Sum3 : Sum  Inputs=-+|
  Transfer Fcn : TransferFcn  Commented=through  Numerator=[L0 R0]  Denominator=[L0/5 R0]
  dq0 to abc : spsdq0toabcLib/dq0 to abc  Alignment=90 degrees behind phase A axis
  dq0 to abc1 : spsdq0toabcLib/dq0 to abc  Alignment=90 degrees behind phase A axis
  upa* : Outport
  una* : Outport  Port=2
  upb* : Outport  Port=3
  unb* : Outport  Port=4
  upc* : Outport  Port=5
  unc* : Outport  Port=6
  wires:
  Product/1 -> dq0 to abc/2
  udiff/1 -> dq0 to abc/1
  ucirc/1 -> dq0 to abc1/1
  Digital Clock/1 -> Product/2, Product1/2
  Gain2/1 -> Product1/1
  Product1/1 -> dq0 to abc1/2
  w/1 -> Product/1, Gain2/1
  Demux/1 -> upa*/1
  Demux/2 -> upb*/1
  Demux/3 -> upc*/1
  Demux1/1 -> una*/1
  Demux1/2 -> unb*/1
  Demux1/3 -> unc*/1
  Sum/1 -> Demux/1
  Sum1/1 -> Demux1/1
  Vdc/1 -> Gain6/1
  dq0 to abc1/1 -> Sum2/1
  Sum2/1 -> Sum/2, Sum1/1
  Gain6/1 -> Sum3/2
  Constant/1 -> Sum3/1
  Sum3/1 -> Mean/1
  Mean/1 -> Transfer Fcn/1
  Transfer Fcn/1 -> Sum2/2, Scope1/1
  dq0 to abc/1 -> Sum1/2, Sum/1

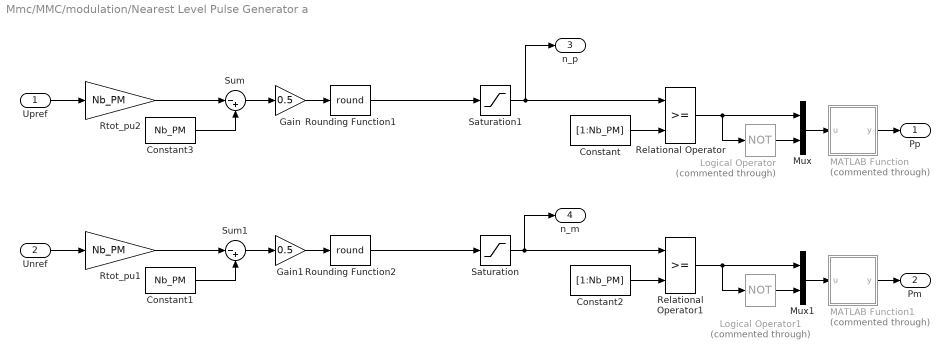
== system Mmc/MMC/modulation/Nearest Level Pulse Generator a  ==
  Upref : Inport
  Unref : Inport  Port=2
  Constant : Constant  Value=[1:Nb_PM]
  Constant1 : Constant  Value=Nb_PM
  Constant2 : Constant  Value=[1:Nb_PM]
  Constant3 : Constant  Value=Nb_PM
  Gain : Gain  Gain=0.5
  Gain1 : Gain  Gain=0.5
  Logical Operator : Logic  Commented=through  Operator=NOT  AllPortsSameDT=off  OutDataTypeStr=float('double')
  Logical Operator1 : Logic  Commented=through  Operator=NOT  AllPortsSameDT=off  OutDataTypeStr=float('double')
  MATLAB Function : MATLAB Function  Commented=through  TreatAsAtomicUnit=on
  MATLAB Function1 : MATLAB Function  Commented=through  TreatAsAtomicUnit=on
  Mux : Mux  Inputs=2
  Mux1 : Mux  Inputs=2
  Relational Operator : RelationalOperator  OutDataTypeStr=float('double')  InputSameDT=off
  Relational Operator1 : RelationalOperator  OutDataTypeStr=float('double')  InputSameDT=off
  Rounding Function1 : Rounding  Operator=round
  Rounding Function2 : Rounding  Operator=round
  Rtot_pu1 : Gain  Gain=Nb_PM  SaturateOnIntegerOverflow=on  OutDataTypeStr=Inherit: Same as input  ParamDataTypeStr=Inherit: Same as input
  Rtot_pu2 : Gain  Gain=Nb_PM  SaturateOnIntegerOverflow=on  OutDataTypeStr=Inherit: Same as input  ParamDataTypeStr=Inherit: Same as input
  Saturation : Saturate  UpperLimit=Nb_PM  LowerLimit=0
  Saturation1 : Saturate  UpperLimit=Nb_PM  LowerLimit=0
  Sum : Sum  Inputs=|-+
  Sum1 : Sum  Inputs=|-+
  Pp : Outport  VectorParamsAs1DForOutWhenUnconnected=off
  Pm : Outport  Port=2  VectorParamsAs1DForOutWhenUnconnected=off
  n_p : Outport  Port=3  VectorParamsAs1DForOutWhenUnconnected=off
  n_m : Outport  Port=4  VectorParamsAs1DForOutWhenUnconnected=off
  wires:
  Constant/1 -> Relational Operator/2
  Relational Operator/1 -> Logical Operator/1, Mux/1
  Logical Operator/1 -> Mux/2
  Mux/1 -> MATLAB Function/1(u)
  MATLAB Function/1(y) -> Pp/1
  Saturation1/1 -> n_p/1, Relational Operator/1
  Rtot_pu2/1 -> Sum/1
  Constant3/1 -> Sum/2
  Sum/1 -> Gain/1
  Gain/1 -> Rounding Function1/1
  Upref/1 -> Rtot_pu2/1
  Constant2/1 -> Relational Operator1/2
  Relational Operator1/1 -> Mux1/1, Logical Operator1/1
  Logical Operator1/1 -> Mux1/2
  Mux1/1 -> MATLAB Function1/1(u)
  MATLAB Function1/1(y) -> Pm/1
  Saturation/1 -> n_m/1, Relational Operator1/1
  Rounding Function1/1 -> Saturation1/1
  Rounding Function2/1 -> Saturation/1
  Sum1/1 -> Gain1/1
  Unref/1 -> Rtot_pu1/1
  Rtot_pu1/1 -> Sum1/1
  Constant1/1 -> Sum1/2
  Gain1/1 -> Rounding Function2/1
